simulink model "feedback_TwoDof"  (R2023b)
settings: Solver=VariableStepAuto  StartTime=0.0  StopTime=10.0  RelTol=1e-3
settings Model: Creator=Egraweb  LastModifiedBy=Egraweb

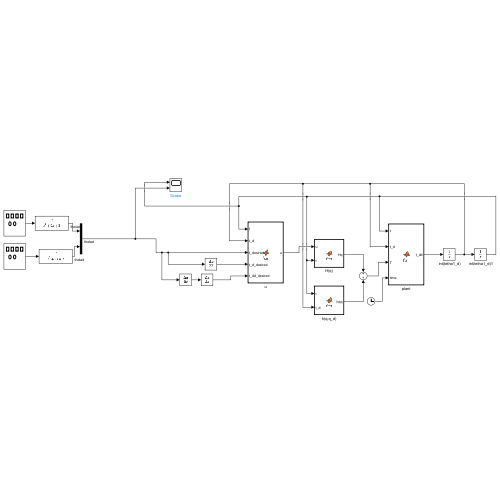
[thumbnail: Simulink's stored preview of the top-level diagram]
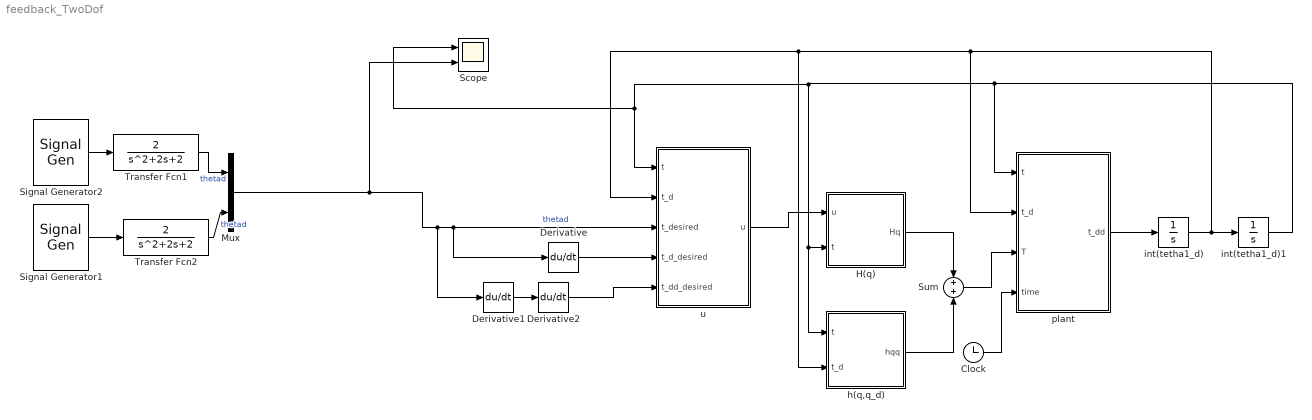
== system feedback_TwoDof ==
  " int(tetha1_d)" : Integrator
  " int(tetha1_d)1" : Integrator
  Clock : Clock
  Derivative : Derivative
  Derivative1 : Derivative
  Derivative2 : Derivative
  H(q) : MATLAB Function  TreatAsAtomicUnit=on
  Mux : Mux  Inputs=2
  Scope : Scope  NumInputPorts=2
  Signal Generator1 : SignalGenerator  Amplitude=2  Frequency=pi  Units=rad/sec
  Signal Generator2 : SignalGenerator  Amplitude=2  Frequency=pi  Units=rad/sec
  Sum : Sum  Inputs=+|+
  Transfer Fcn1 : TransferFcn  Numerator=[2]  Denominator=[1 2 2]
  Transfer Fcn2 : TransferFcn  Numerator=[2]  Denominator=[1 2 2]
  h(q,q_d) : MATLAB Function  TreatAsAtomicUnit=on
  plant : MATLAB Function  TreatAsAtomicUnit=on
  u : MATLAB Function  TreatAsAtomicUnit=on
  wires:
  plant/1(t_dd) -> " int(tetha1_d)"/1
  " int(tetha1_d)"/1 -> plant/2(t_d), u/2(t_d), h(q,q_d)/2(t_d), " int(tetha1_d)1"/1
  " int(tetha1_d)1"/1 -> plant/1(t), Scope/1, u/1(t), h(q,q_d)/1(t), H(q)/2(t)
  H(q)/1(Hq) -> Sum/1
  h(q,q_d)/1(hqq) -> Sum/2
  Sum/1 -> plant/3(T)
  u/1(u) -> H(q)/1(u)
  Derivative/1 -> u/4(t_d_desired)
  Derivative1/1 -> Derivative2/1
  Derivative2/1 -> u/5(t_dd_desired)
  Signal Generator1/1 -> Transfer Fcn2/1
  Transfer Fcn1/1 -> Mux/1  "thetad"
  Transfer Fcn2/1 -> Mux/2  "thetad"
  Signal Generator2/1 -> Transfer Fcn1/1
  Mux/1 -> Derivative1/1, Derivative/1, u/3(t_desired), Scope/2  "thetad"
  Clock/1 -> plant/4(time)

== matlab function feedback_TwoDof/H(q) ==
  data: u input; Hq output; t input
function Hq = fcn(u, t)
Hq=[0;0];
m1 = 1;
m2 = 1;
l1 = 1;
lc1 = 0.5;
l2 = 1;
lc2 = 0.5;
g = 9.81;

H11 = m1*lc1^2 + l1 + m2*(l1^2+lc2^2+2*l1*lc2*cos(t(2)))+l2;
H22 = m2*lc2^2 + l2;
H12 = m2*l1*lc2*cos(t(2)) + m2*lc2^2 + l2;
H21 = m2*l1*lc2*cos(t(2)) + m2*lc2^2 + l2;

H = [H11 H12; H21 H22];

Hq = H*u;

== matlab function feedback_TwoDof/plant ==
  data: t input; t_dd output; t_d input; T input; time input
function t_dd = fcn(t, t_d, T , time)

t_dd =[0;0];

d = 20 * sin(pi*time);

m1 = 1;
m2 = 1;
l1 = 1;
lc1 = 0.5;
l2 = 1;
lc2 = 0.5;
g = 9.81;

H11 = m1*lc1^2 + l1 + m2*(l1^2+lc2^2+2*l1*lc2*cos(t(2)))+l2;
H22 = m2*lc2^2 + l2;
H12 = m2*l1*lc2*cos(t(2)) + m2*lc2^2 + l2;
H21 = m2*l1*lc2*cos(t(2)) + m2*lc2^2 + l2;

H = [H11 H12; H21 H22];
h = m2*l1*lc2*sin(t(2));
g1 = m1*lc1*g*cos(t(1)) + m2*g*(lc2*cos(t(1)+t(2))+l1*cos(t(1)));
g2 = m2*lc2*g*cos(t(1)+t(2));
t_dd = inv(H)*(T - [-h*t_d(2) -h*t_d(1)-h*t_d(2); h*t_d(1) 0]*[t_d(1); t_d(2)]-[g1; g2] + d);

== matlab function feedback_TwoDof/h(q,q_d) ==
  data: t input; hqq output; t_d input
function hqq = fcn(t, t_d)

hqq = [0;0];
t1=t(1);
t2=t(2);
t_d1=t_d(1);
t_d2=t_d(2);

m1 = 1;
m2 = 1;
l1 = 1;
lc1 = 0.5;
l2 = 1;
lc2 = 0.5;
h = m2*l1*lc2*sin(t(2));
g = 9.81;

g1 = m1*lc1*g*cos(t1) + m2*g*(lc2*cos(t1+t2)+l1*cos(t1));
g2 = m2*lc2*g*cos(t1+t2);

hqq = [-h*t_d2 -h*t_d1-h*t_d2; h*t_d1 0]*[t_d1; t_d2]+[g1; g2];

== matlab function feedback_TwoDof/u ==
  data: t input; u output; t_d input; t_desired input; t_d_desired input; t_dd_desired input
function u = fcn(t, t_d, t_desired, t_d_desired, t_dd_desired)

KD = 20;
KP = 100;
tetha_tilted = t - t_desired;
tetha_d_tilted = t_d - t_d_desired;
u = t_dd_desired-(KD*(tetha_d_tilted))-(KP*(tetha_tilted));
